simulink model "Peregrine_falcon_in_still_flight_model"  (R2025b)
settings: Solver=VariableStepAuto  StartTime=0.0  StopTime=5  RelTol=1e-3
undefined symbols (not defined in the file): A, Cd, g, m, rho
settings Model: Creator=User  LastModifiedBy=User

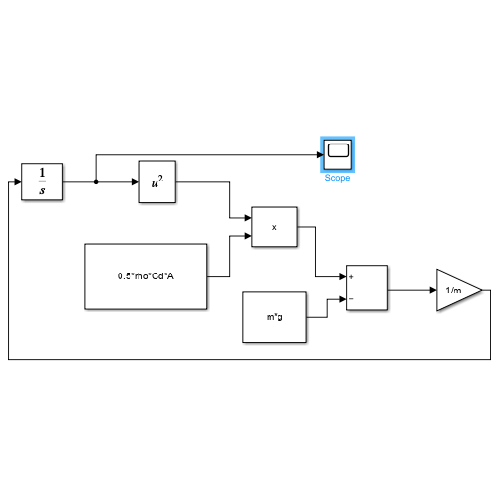
[thumbnail: Simulink's stored preview of the top-level diagram]
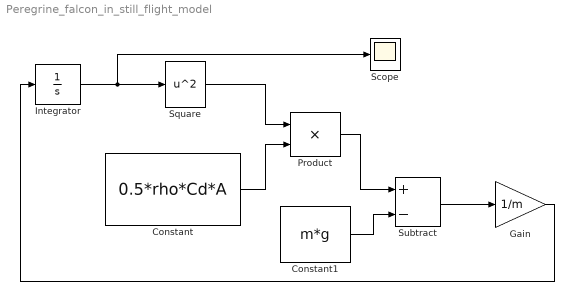
== system Peregrine_falcon_in_still_flight_model ==
  Constant : Constant  Value=0.5*rho*Cd*A
  Constant1 : Constant  Value=m*g
  Gain : Gain  Gain=1/m
  Integrator : Integrator
  Product : Product
  Scope : Scope
      settings: ActiveDisplayYMinimum=-52.016420784234661  ActiveDisplayYMaximum=5.7796023093594062
  Square : Math  Operator=square
  Subtract : Sum  Inputs=+-
  wires:
  Integrator/1 -> Scope/1, Square/1
  Square/1 -> Product/1
  Constant/1 -> Product/2
  Product/1 -> Subtract/1
  Constant1/1 -> Subtract/2
  Subtract/1 -> Gain/1
  Gain/1 -> Integrator/1
